simulink model "Mobileye630_V"  (R2021a)
settings: Solver=VariableStepAuto  StartTime=0.0  StopTime=100  RelTol=1e-3
undefined symbols (not defined in the file): canChannel
libraries: canlib x2, canmsglib x1
settings Model: EnablePacing=on  Creator=sgttr  LastModifiedBy=sgttr

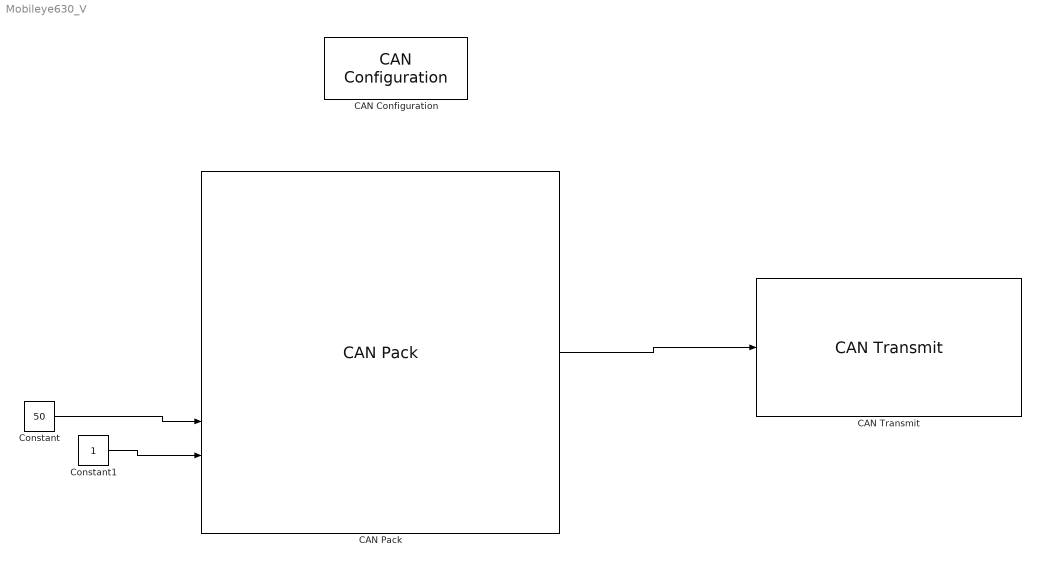
== system Mobileye630_V ==
  CAN Configuration : canlib/CAN Configuration  BlockHandle=2.0002  Device=MathWorks Virtual 1 (Channel 1)  DeviceMenu=MathWorks Virtual 1 (Channel 1)  ObjConstructor=canChannel('MathWorks', 'Virtual 1', 1)  BusSpeed=500000  EnableBitParameters=off  AckMode=Normal
      settings: SourceProductBaseCode=VN
  CAN Pack : canmsglib/CAN Pack  CANdbFile=D:\ADAS-Camera-hardware-in-the-loop-testing-master\Current process of Mobileye 630\Mobileye.dbc  MsgList=Vehicle_State  MsgName=Vehicle_State  MsgIDType=Standard (11-bit identifier)  MsgIdentifier=1888  MsgLength=8  Remote=off  ApplyMinMax=off  BusOutput=off  SignalInfo={ 'Brake_Signal', '0', '1', 'LE', 'unsigned', 'Standard', '0', '1', '0', '0', '1'; 'High_Beam', '5', '1', 'LE', 'unsigned', 'Standard', '0', '1', '0', '0', '1'; 'High_Beam_Available', '13', '1', 'LE', 'unsigned', 'Standard', '0', '1', '0', '0', '1'; 'Left_Signal', '1', '1', 'LE', 'unsigned', 'Standard', '0', '1', '0', '0', '1'; 'Low_Beam', '4', '1', 'LE', 'unsigned', 'Standard', '0', '1', '0', '0', '1'; 'Low_Beam_Available', '12', '1', 'LE', 'unsigned', 'Standard', '0', '1', '0', '0', '1'; 'Right_Signal', '2', '1', 'LE', 'unsigned', 'Standard', '0', '1', '0', '0', '1'; 'Speed', '16', '8', 'LE', 'unsigned', 'Standard', '0', '1', '0', '0', '255'; 'Speed_Available', '15', '1', 'LE', 'unsigned', 'Standard', '0', '1', '0', '0', '1'; 'Wipers', '3', '1', 'LE', 'unsigned', 'Standard', '0', '1', '0', '0', '1'; 'Wipers_Available', '11', '1', 'LE', 'unsigned', 'Standard', '0', '1', '0', '0', '1' }
      settings: SourceProductBaseCode=ME,XP,VN  DataFormat=CANdb specified signals
  CAN Transmit : canlib/CAN Transmit  BlockHandle=4.0002  Device=MathWorks Virtual 1 (Channel 1)  DeviceMenu=MathWorks Virtual 1 (Channel 1)  ObjConstructor=canChannel('MathWorks', 'Virtual 1', 1)  EnableEventTransmit=off  EnablePeriodicTransmit=off  MessagePeriod=1.000
      settings: SourceProductBaseCode=VN
  Constant : Constant  Value=50  SampleTime=0.015
  Constant1 : Constant  SampleTime=0.015
  wires:
  CAN Pack/1 -> CAN Transmit/1
  Constant/1 -> CAN Pack/8
  Constant1/1 -> CAN Pack/9
